simulink model "motorcc"  (R2024a)
settings: Solver=VariableStepAuto  StartTime=0.0  StopTime=5  RelTol=1e-3
values from neighbouring files (symbols this model uses):
  Bm = 4.48491e-6    (= 4.48491e-06)    [projeto_controlador_pi.m]
  Jm = 2.03448e-5    (= 2.03448e-05)    [projeto_controlador_pi.m]
  Ke = 0.009530212    [projeto_controlador_pi.m]
  Ki = 30.3    [projeto_controlador_pi.m]
  Kp = 1    [projeto_controlador_pi.m]
  Kt = 0.009737475    [projeto_controlador_pi.m]
  Ktaco = 0.0035014    [projeto_controlador_pi.m]
  La = 94.87e-6    (= 9.487e-05)    [projeto_controlador_pi.m]
  Ra = 0.158109983    [projeto_controlador_pi.m]
  Tc = 0.006683397    [projeto_controlador_pi.m]
libraries: slpidlib x1
settings Model: Creator=franc  LastModifiedBy=franc
settings RTWCC: GPUComputeCapability=3.5

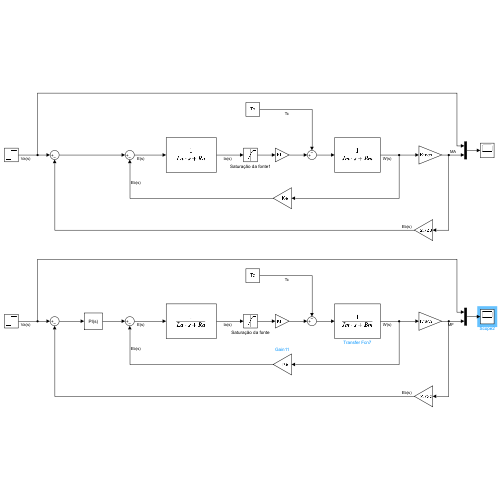
[thumbnail: Simulink's stored preview of the top-level diagram]
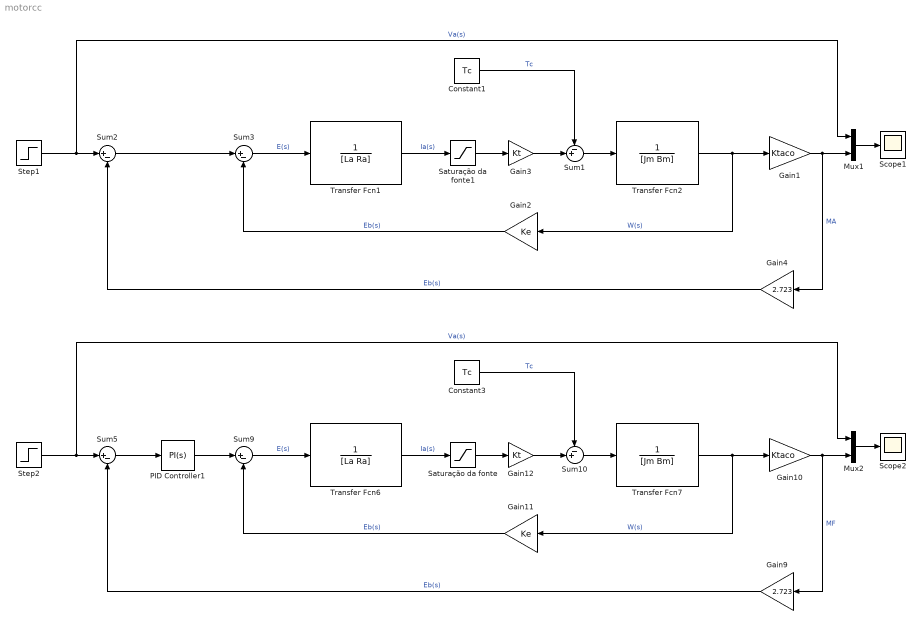
== system motorcc ==
  Constant1 : Constant  Value=Tc  VectorParams1D=off
  Constant3 : Constant  Value=Tc  VectorParams1D=off
  Gain1 : Gain  Gain=Ktaco
  Gain10 : Gain  Gain=Ktaco
  Gain11 : Gain  Gain=Ke
  Gain12 : Gain  Gain=Kt
  Gain2 : Gain  Gain=Ke
  Gain3 : Gain  Gain=Kt
  Gain4 : Gain  Gain=2.723
  Gain9 : Gain  Gain=2.723
  Mux1 : Mux  Inputs=2
  Mux2 : Mux  Inputs=2
  PID Controller1 : slpidlib/PID Controller  Controller=PI  Form=Parallel  TimeDomain=Continuous-time  UseExternalTs=off  SampleTime=-1  IntegratorMethod=Forward Euler  FilterMethod=Forward Euler  ControllerParametersSource=internal  P=Kp  I=Ki  UseKiTs=off  D=0.000316  UseExternalDerivativeSource=off  N=100  UseFilter=on  TunerSelectOption=Transfer Function Based (PID Tuner App)  InitialConditionSource=internal  InitialConditionForIntegrator=0  InitialConditionForFilter=0  DifferentiatorICPrevScaledInput=0  ExternalReset=none  TrackingMode=off  Kt=1  LimitOutput=off  SatLimitsSource=internal  UpperSaturationLimit=inf  LowerSaturationLimit=-inf  LinearizeAsGain=on  AntiWindupMode=none  Kb=1  LimitIntegrator=off  UpperIntegratorSaturationLimit=inf  LowerIntegratorSaturationLimit=-inf  POutMin=[]  POutMax=[]  IOutMin=[]  IOutMax=[]  DOutMin=[]  DOutMax=[]  NOutMin=[]  NOutMax=[]  SumOutMin=[]  SumOutMax=[]  SaturationOutMin=[]  SaturationOutMax=[]  PParamMin=[]  PParamMax=[]  IParamMin=[]  IParamMax=[]  DParamMin=[]  DParamMax=[]  NParamMin=[]  NParamMax=[]  KbParamMin=[]  KbParamMax=[]  KtParamMin=[]  KtParamMax=[]  KbOutMin=[]  KbOutMax=[]  KtOutMin=[]  KtOutMax=[]  IntegratorOutMin=[]  IntegratorOutMax=[]  FilterOutMin=[]  FilterOutMax=[]  SumI1OutMin=[]  SumI1OutMax=[]  SumI2OutMin=[]  SumI2OutMax=[]  SumI3OutMin=[]  SumI3OutMax=[]  SumI4OutMin=[]  SumI4OutMax=[]  SumDOutMin=[]  SumDOutMax=[]  DifferentiatorOutMin=[]  DifferentiatorOutMax=[]  FilterDiffOutCoefMin=[]  FilterDiffOutCoefMax=[]  ReciprocalOutMin=[]  ReciprocalOutMax=[]  SumDenOutMin=[]  SumDenOutMax=[]  SumNumOutMin=[]  SumNumOutMax=[]  DivideOutMin=[]  DivideOutMax=[]  UdiffTsProdOutMin=[]  UdiffTsProdOutMax=[]  NTsProdOutMin=[]  NTsProdOutMax=[]  UintegralTsProdOutMin=[]  UintegralTsProdOutMax=[]  UngainTsProdOutMin=[]  UngainTsProdOutMax=[]  ClampingZeroOutDataTypeStr=Inherit: Inherit via back propagation  ClampingZeroOutMin=[]  ClampingZeroOutMax=[]  FilterDenConstantOutDataTypeStr=Inherit: Inherit via back propagation  FilterDenConstantOutMin=[]  FilterDenConstantOutMax=[]  PCopyOutDataTypeStr=Inherit: Inherit via back propagation  PCopyOutMin=[]  PCopyOutMax=[]  NCopyOutDataTypeStr=Inherit: Inherit via back propagation  NCopyOutMin=[]  NCopyOutMax=[]  IntegratorContinuousStateAttributes=''  IntegratorStateMustResolveToSignalObject=off  IntegratorRTWStateStorageClass=Auto  FilterContinuousStateAttributes=''  FilterStateMustResolveToSignalObject=off  FilterRTWStateStorageClass=Auto  ParallelPVariant=InternalParameters  IdealPVariant=Disabled  IVariant=InternalParameters  DVariant=Disabled  IntegratorVariant=Continuous  SatVariant=Disabled  AWVariant=Passthrough  PCopyVariant=Disabled  TRVariant=Disabled  FdbkBlocksVariant=Forward  IdealPFdbkVariant=Disabled  SatFdbkVariant=Disabled  DerivativeFilterVariant=Disabled  NVariant=Disabled  NCopyVariant=Disabled_SignalSpec  FilterICVariant=Disabled  IntegratorICVariant=InternalICs  ExternalResetVariant=Disabled  TRSumVariant=Passthrough  SumFdbkVariant=Disabled  SumVariant=Sum_PI  TsampFilterVariant=InternalTs  TsampNgainVariant=Passthrough  TsampIntegralVariant=Disabled_SignalSpec  ExternalSaturationOutDataTypeStr=Inherit: Same as second input  DerivativeSourceVariant=Disabled
  Saturação da fonte : Saturate  UpperLimit=22  LowerLimit=-22
  Saturação da fonte1 : Saturate  UpperLimit=22  LowerLimit=-22
  Scope1 : Scope
  Scope2 : Scope
  Step1 : Step  After=12  SampleTime=0  VectorParams1D=off  ZeroCross=off
  Step2 : Step  After=12  SampleTime=0
  Sum1 : Sum  Inputs=-+|
  Sum10 : Sum  Inputs=-+|
  Sum{2..3,5,9} (4 alike) : Sum  Inputs=|+-
  Transfer Fcn1 : TransferFcn  Denominator=[La Ra]
  Transfer Fcn2 : TransferFcn  Denominator=[Jm Bm]
  Transfer Fcn6 : TransferFcn  Denominator=[La Ra]
  Transfer Fcn7 : TransferFcn  Denominator=[Jm Bm]
  wires:
  Gain12/1 -> Sum10/2
  Sum9/1 -> Transfer Fcn6/1  "E(s)"
  Sum10/1 -> Transfer Fcn7/1
  Constant3/1 -> Sum10/1  "Tc"
  Mux2/1 -> Scope2/1
  Gain10/1 -> Gain9/1, Mux2/2  "MF"
  Gain11/1 -> Sum9/2  "Eb(s)"
  Transfer Fcn7/1 -> Gain11/1, Gain10/1  "W(s)"
  Transfer Fcn6/1 -> Saturação da fonte/1  "Ia(s)"
  Gain9/1 -> Sum5/2  "Eb(s)"
  Sum5/1 -> PID Controller1/1
  PID Controller1/1 -> Sum9/1
  Saturação da fonte/1 -> Gain12/1
  Step2/1 -> Sum5/1, Mux2/1  "Va(s)"
  Step1/1 -> Sum2/1, Mux1/1  "Va(s)"
  Saturação da fonte1/1 -> Gain3/1
  Mux1/1 -> Scope1/1
  Sum2/1 -> Sum3/1
  Gain1/1 -> Gain4/1, Mux1/2  "MA"
  Gain4/1 -> Sum2/2  "Eb(s)"
  Sum3/1 -> Transfer Fcn1/1  "E(s)"
  Transfer Fcn2/1 -> Gain2/1, Gain1/1  "W(s)"
  Gain2/1 -> Sum3/2  "Eb(s)"
  Sum1/1 -> Transfer Fcn2/1
  Transfer Fcn1/1 -> Saturação da fonte1/1  "Ia(s)"
  Gain3/1 -> Sum1/2
  Constant1/1 -> Sum1/1  "Tc"
